simulink model "Lab2_6"  (Simulink 7.3)
settings: Solver=ode45  StartTime=3.0  StopTime=10.0  RelTol=1e-3
libraries: simulink x2
settings Model: Creator=Seva  LastModifiedBy=Seva

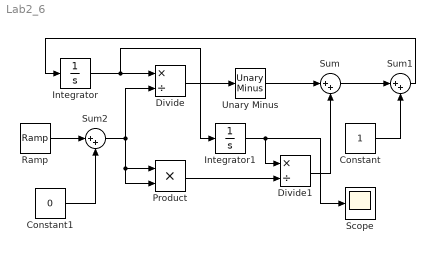
== system Lab2_6 ==
  Constant : Constant  OutDataType=fixdt(1, 16)  OutScaling=2^0
  Constant1 : Constant  Value=0  OutDataType=fixdt(1, 16)  OutScaling=2^0
  Divide : Product  Inputs=*/  OutDataType=fixdt(1, 16)  OutScaling=2^-10
  Divide1 : Product  Inputs=*/  OutDataType=fixdt(1, 16)  OutScaling=2^-10
  Integrator : Integrator  InitialCondition=3
  Integrator1 : Integrator  InitialCondition=6
  Product : Product  OutDataType=fixdt(1, 16)  OutScaling=2^0  RndMeth=Zero
  Ramp : simulink/Sources/Ramp  SystemSampleTime=-1  slope=1  start=0  X0=0
  Scope : Scope
  Sum : Sum  Inputs=|++  OutDataType=fixdt(1, 16)  OutScaling=2^0
  Sum1 : Sum  Inputs=|++  OutDataType=fixdt(1, 16)  OutScaling=2^0
  Sum2 : Sum  Inputs=|++  OutDataType=fixdt(1, 16)  OutScaling=2^0
  Unary Minus : simulink/Math Operations/Unary Minus  DoSatur=off
  wires:
  Divide/1 -> Unary Minus/1
  Integrator/1 -> Divide/1, Integrator1/1
  Product/1 -> Divide1/2
  Integrator1/1 -> Divide1/1, Scope/1
  Unary Minus/1 -> Sum/1
  Divide1/1 -> Sum/2
  Constant/1 -> Sum1/2
  Sum/1 -> Sum1/1
  Sum1/1 -> Integrator/1
  Ramp/1 -> Sum2/1
  Constant1/1 -> Sum2/2
  Sum2/1 -> Divide/2, Product/1, Product/2
